simulink model "Test_Decoder_4_to_16"  (Simulink 8.1)
settings: Solver=ode45  StartTime=0.0  StopTime=len  RelTol=1e-3
libraries: commutil2 x2, Decoders_Lib x1
settings Model: Creator=N  LastModifiedBy=uzivatel
settings DataIOCC: LimitDataPoints=off  SignalLoggingSaveFormat=Dataset
settings OptimizationCC: ExpressionDepthLimit=128
settings DebuggingCC: UnderspecifiedInitializationDetection=Simplified  MergeDetectMultiDrivingBlocksExec=error  SolverPrmCheckMsg=none  FcnCallInpInsideContextMsg=EnableAllAsError  FrameProcessingCompatibilityMsg=error  StateNameClashWarn=none
settings HardwareCC: ProdBitPerPointer=64  ProdLargestAtomicFloat=Float  ProdIntDivRoundTo=Zero  ProdEndianess=LittleEndian  ProdHWDeviceType=Intel->x86-64 (Windows64)
settings ModelReferenceCC: PropagateSignalLabelsOutOfModel=on
settings GRTTargetCC: CodeReplacementLibrary=None  CombineOutputUpdateFcns=on  CPPClassGenCompliant=on  GRTInterface=off

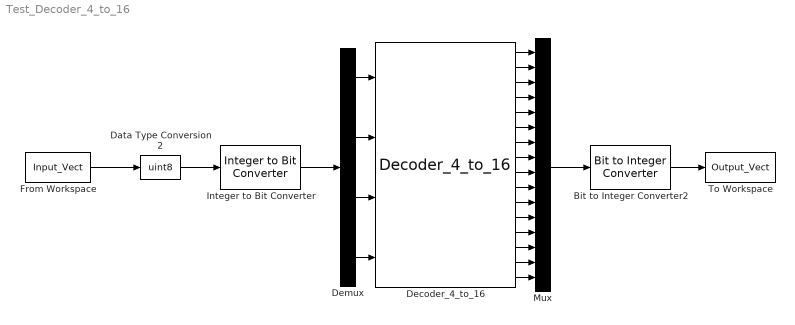
== system Test_Decoder_4_to_16 ==
  Bit to Integer Converter2 : commutil2/Bit to Integer Converter  nbits=16  bitOrder=MSB first  signedOutputValues=Unsigned  outDtype=uint16  outDtypeSigned=Inherit via internal rule
  Data Type Conversion2 : DataTypeConversion  OutDataTypeStr=uint8
  Decoder_4_to_16 : Decoders_Lib/Decoders_Lib/Decoder_4_to_16
  Demux : Demux
  From Workspace : FromWorkspace  VariableName=Input_Vect  SampleTime=1  Interpolate=off  OutputAfterFinalValue=Holding final value
  Integer to Bit Converter : commutil2/Integer to Bit Converter  nbits=4  signedInputValues=Unsigned  bitOrder=MSB first  outDtype=uint8
  Mux : Mux  Inputs=16
  To Workspace : ToWorkspace  VariableName=Output_Vect  SampleTime=1
  wires:
  Decoder_4_to_16/1 -> Mux/1
  Decoder_4_to_16/2 -> Mux/2
  Decoder_4_to_16/3 -> Mux/3
  Decoder_4_to_16/4 -> Mux/4
  Decoder_4_to_16/5 -> Mux/5
  Decoder_4_to_16/6 -> Mux/6
  Decoder_4_to_16/7 -> Mux/7
  Decoder_4_to_16/8 -> Mux/8
  Decoder_4_to_16/9 -> Mux/9
  Decoder_4_to_16/10 -> Mux/10
  Decoder_4_to_16/11 -> Mux/11
  Decoder_4_to_16/12 -> Mux/12
  Decoder_4_to_16/13 -> Mux/13
  Decoder_4_to_16/14 -> Mux/14
  Decoder_4_to_16/15 -> Mux/15
  Decoder_4_to_16/16 -> Mux/16
  Demux/1 -> Decoder_4_to_16/1
  Demux/2 -> Decoder_4_to_16/2
  Demux/3 -> Decoder_4_to_16/3
  Demux/4 -> Decoder_4_to_16/4
  Integer to Bit Converter/1 -> Demux/1
  Data Type Conversion2/1 -> Integer to Bit Converter/1
  Mux/1 -> Bit to Integer Converter2/1
  From Workspace/1 -> Data Type Conversion2/1
  Bit to Integer Converter2/1 -> To Workspace/1
